simulink model "states"  (R2020b)
settings: Solver=FixedStepDiscrete  StartTime=0.0  StopTime=60.0  FixedStep=0.1  RelTol=1e-3  EnableMultiTasking=on
settings Model: Creator=ana  LastModifiedBy=ana
settings SolverCC: AutoInsertRateTranBlk=on
settings OptimizationCC: LifeSpan=inf
settings DebuggingCC: SFUnexpectedBacktrackingDiag=warning  SFNoUnconditionalDefaultTransitionDiag=warning  SFExecutionAtInitializationDiag=none  ArithmeticOperatorsInVariantConditions=warning
settings SFSimCC: SimUseLocalCustomCode=off  CustomCodeUndefinedFunction=UseInterfaceOnly
settings RTWCC: RTWUseLocalCustomCode=off
settings CodeAppCC: StateflowObjectComments=on
settings GRTTargetCC: TargetLangStandard=C89/C90 (ANSI)
settings ConfigComp: CovMetricSettings=dw  CovSaveCumulativeToWorkspaceVar=on  CovSaveSingleToWorkspaceVar=on  CovExternalEMLEnable=off

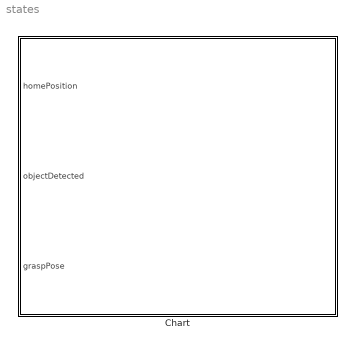
== system states ==
  Chart : Stateflow chart  TreatAsAtomicUnit=on

== stateflow chart states/Chart ==
  state DetectObject
    % detect ocject with sensors and pass on coordinates and
    % mass center
  state HomePosition
    entry:
    homePosition;
    % robot coordinates as input from environment
    % periodically check if there are any objects to be picked up
  state Execute
    entry: objectPicked = false; objectPlaced = false; graspPose;
    state Pick
      state ComputeGraspPose
        % need the center of mass
        % and the top of the object
      state MoveToReachPosition
        % move from current home
        % position to the grasp pose
      state PickUpObject
        % activate gripper
      state MoveToRetractedPosition
        % move from grasp pose to
        % retracted position
        exit:
        objectPicked = true;
      (default) -> ComputeGraspPose
      ComputeGraspPose -> MoveToReachPosition
      MoveToReachPosition -> PickUpObject
      PickUpObject -> Execute.Pick.MoveToRetractedPosition
    state Place
      state PlaceObject
        % deactivate gripper
      state ComputePlacementPosition
        % call placement algorithm to
        % get position
      state MoveToPlacementPosition
        % move from current retracted
        % position to the placement pose
      state MoveToRetractedPosition
        % move from current placement
        % position to the retracted pose
        exit:
        % move from current retracted
        % position to the home position
      (default) -> ComputePlacementPosition
      MoveToPlacementPosition -> PlaceObject
      PlaceObject -> Execute.Place.MoveToRetractedPosition
      ComputePlacementPosition -> MoveToPlacementPosition
    (default) -> Pick
    Pick -> Place : [objectPicked]
  (default) -> HomePosition
  HomePosition -> DetectObject : after(3, sec)
  Place -> HomePosition : [objectPlaced]
  DetectObject -> HomePosition [order 2] : [~objectDetected]
  DetectObject -> Execute [order 1] : [objectDetected]
  data: homePosition input; objectPicked local; objectPlaced local; objectDetected input; graspPose input
